simulink model "diff_drive_sim"  (Simulink 10.3)
settings: Solver=VariableStepAuto  StartTime=0.0  StopTime=30.1  RelTol=1e-3
values from neighbouring files (symbols this model uses):
  a = 4    [diff_drive.m]
  d = 0.1    [diff_drive.m]
  Kp = 1    [diff_drive.m]
  Kth = 2    [diff_drive.m]
  Kx = 15    [diff_drive.m]
  Ky = 15    [diff_drive.m]
  theta0 = pi/2    (= 1.57079632679)    [diff_drive.m]
  w = 0.1    [diff_drive.m]
  x0 = a    (= 4)    [diff_drive.m]
  y0 = 0    [diff_drive.m]
settings Model: Creator=olivier  LastModifiedBy=yukisaito  MultithreadedSim=on
settings SolverCC: ZeroCrossAlgorithm=Adaptive
settings DataIOCC: SaveFormat=Dataset  SignalLoggingSaveFormat=Dataset
settings OptimizationCC: ExpressionDepthLimit=128  LifeSpan=auto
settings DebuggingCC: UnderspecifiedInitializationDetection=Simplified  MergeDetectMultiDrivingBlocksExec=error  MaskedZcDiagnostic=none  IgnoredZcDiagnostic=none  FcnCallInpInsideContextMsg=error  StateNameClashWarn=none  SFUnexpectedBacktrackingDiag=error  SFNoUnconditionalDefaultTransitionDiag=error  SFExecutionAtInitializationDiag=warning
settings HardwareCC: ProdBitPerPointer=64  ProdBitPerSizeT=64  ProdBitPerPtrDiffT=64  ProdLargestAtomicFloat=Float  ProdIntDivRoundTo=Zero  ProdEndianess=LittleEndian  ProdWordSize=64  ProdHWDeviceType=Intel->x86-64 (Windows64)
settings ModelReferenceCC: PropagateSignalLabelsOutOfModel=on
settings SFSimCC: SimUseLocalCustomCode=on
settings RTWCC: RTWUseLocalCustomCode=on
settings CodeAppCC: StateflowObjectComments=off
settings GRTTargetCC: TargetLangStandard=C99 (ISO)  CombineOutputUpdateFcns=on  GRTInterface=off
settings ConfigComp: CovMetricSettings=dwe  CovSaveCumulativeToWorkspaceVar=off  CovSaveSingleToWorkspaceVar=off  CovExternalEMLEnable=on

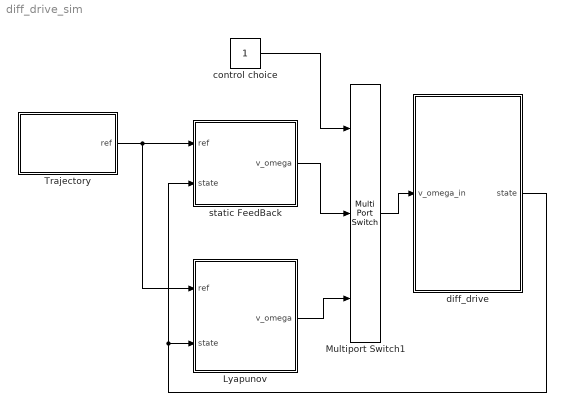
== system diff_drive_sim ==
  Lyapunov : Subsystem
  Multiport Switch1 : MultiPortSwitch  Inputs=2
  Trajectory : Subsystem  TreatAsAtomicUnit=on
  control choice : Constant
  diff_drive : Subsystem  mask{base=0.5, base_error=0, radius=0.2, radius_error=0, omega_max=80}
      mask prompts: base_error "Base error in percent"; radius_error "Radius error in percent"; omega_max "Wheel Max Velocity"
  static FeedBack : Subsystem
  wires:
  Trajectory/1(ref) -> Lyapunov/1(ref), static FeedBack/1(ref)
  Multiport Switch1/1 -> diff_drive/1(v_omega_in)
  control choice/1 -> Multiport Switch1/1
  diff_drive/1(state) -> static FeedBack/2(state), Lyapunov/2(state)
  static FeedBack/1(v_omega) -> Multiport Switch1/2
  Lyapunov/1(v_omega) -> Multiport Switch1/3

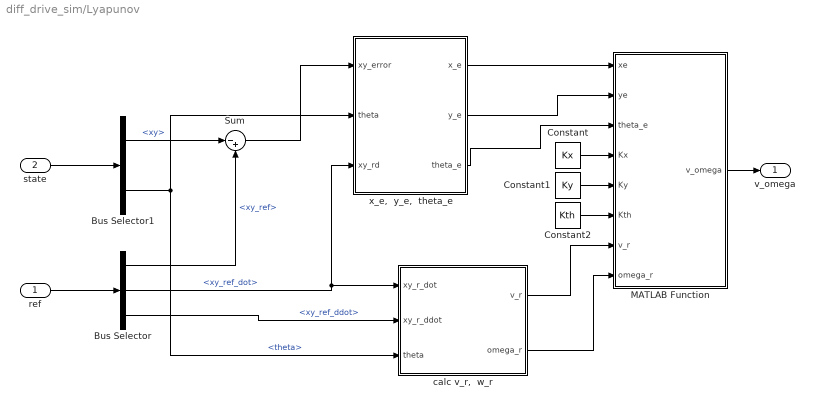
== system diff_drive_sim/Lyapunov ==
  ref : Inport
  state : Inport  Port=2
  Bus Selector : BusSelector  OutputSignals=xy_ref,xy_ref_dot,xy_ref_ddot
  Bus Selector1 : BusSelector  OutputSignals=xy,theta
  Constant : Constant  Value=Kx  VectorParams1D=off
  Constant1 : Constant  Value=Ky
  Constant2 : Constant  Value=Kth
  MATLAB Function : MATLAB Function  TreatAsAtomicUnit=on
  Sum : Sum  Inputs=|-+
  "calc v_r,  w_r" : MATLAB Function  TreatAsAtomicUnit=on
  "x_e,  y_e,  theta_e" : MATLAB Function  TreatAsAtomicUnit=on
  v_omega : Outport  VectorParamsAs1DForOutWhenUnconnected=off
  wires:
  ref/1 -> Bus Selector/1
  state/1 -> Bus Selector1/1
  Bus Selector/2 -> "x_e,  y_e,  theta_e"/3(xy_rd), "calc v_r,  w_r"/1(xy_r_dot)  "<xy_ref_dot>"
  Bus Selector/1 -> Sum/2  "<xy_ref>"
  Bus Selector/3 -> "calc v_r,  w_r"/2(xy_r_ddot)  "<xy_ref_ddot>"
  Bus Selector1/1 -> Sum/1  "<xy>"
  Bus Selector1/2 -> "x_e,  y_e,  theta_e"/2(theta), "calc v_r,  w_r"/3(theta)  "<theta>"
  Sum/1 -> "x_e,  y_e,  theta_e"/1(xy_error)
  MATLAB Function/1(v_omega) -> v_omega/1
  "x_e,  y_e,  theta_e"/1(x_e) -> MATLAB Function/1(xe)
  "x_e,  y_e,  theta_e"/2(y_e) -> MATLAB Function/2(ye)
  "x_e,  y_e,  theta_e"/3(theta_e) -> MATLAB Function/3(theta_e)
  "calc v_r,  w_r"/1(v_r) -> MATLAB Function/7(v_r)
  "calc v_r,  w_r"/2(omega_r) -> MATLAB Function/8(omega_r)
  Constant1/1 -> MATLAB Function/5(Ky)
  Constant/1 -> MATLAB Function/4(Kx)
  Constant2/1 -> MATLAB Function/6(Kth)

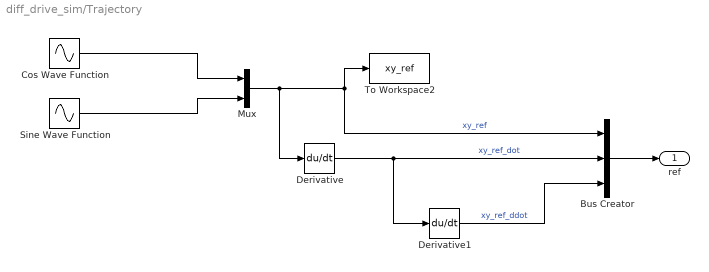
== system diff_drive_sim/Trajectory ==
  Bus Creator : BusCreator  Inputs=3
  Cos Wave Function : Sin  Amplitude=a  Frequency=w  Phase=pi/2  SampleTime=0
  Derivative : Derivative
  Derivative1 : Derivative
  Mux : Mux  Inputs=2
  Sine Wave Function : Sin  Amplitude=a  Frequency=w  SampleTime=0
  To Workspace2 : ToWorkspace  VariableName=xy_ref  SampleTime=-1
      settings: Save2DSignal=2-D array (concatenate along first dimension)
  ref : Outport  VectorParamsAs1DForOutWhenUnconnected=off
  wires:
  Bus Creator/1 -> ref/1
  Mux/1 -> Derivative/1, Bus Creator/1, To Workspace2/1  "xy_ref"
  Derivative/1 -> Bus Creator/2, Derivative1/1  "xy_ref_dot"
  Derivative1/1 -> Bus Creator/3  "xy_ref_ddot"
  Sine Wave Function/1 -> Mux/2
  Cos Wave Function/1 -> Mux/1

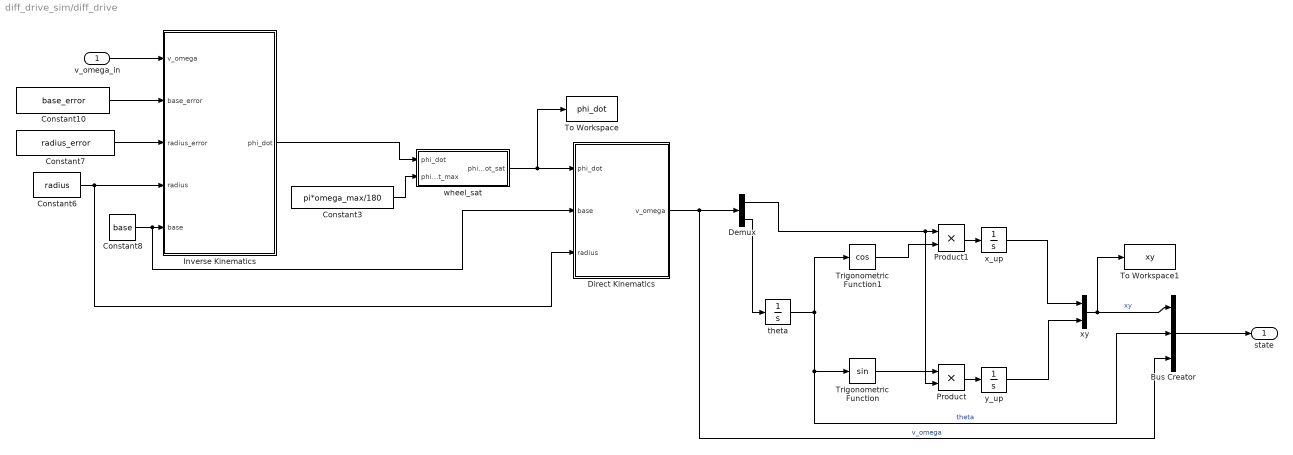
== system diff_drive_sim/diff_drive ==
  v_omega_in : Inport
  Bus Creator : BusCreator  Inputs=3
  Constant10 : Constant  Value=base_error
  Constant3 : Constant  Value=pi*omega_max/180
  Constant6 : Constant  Value=radius
  Constant7 : Constant  Value=radius_error
  Constant8 : Constant  Value=base
  Demux : Demux  Outputs=2
  Direct Kinematics : MATLAB Function  TreatAsAtomicUnit=on
  Inverse Kinematics : MATLAB Function  TreatAsAtomicUnit=on
  Product : Product
  Product1 : Product
  To Workspace : ToWorkspace  VariableName=phi_dot  SampleTime=-1
      settings: Save2DSignal=2-D array (concatenate along first dimension)
  To Workspace1 : ToWorkspace  VariableName=xy  SampleTime=-1
      settings: Save2DSignal=2-D array (concatenate along first dimension)
  Trigonometric Function : Trigonometry
  Trigonometric Function1 : Trigonometry  Operator=cos
  theta : Integrator  InitialCondition=theta0
  wheel_sat : Subsystem
  x_up : Integrator  InitialCondition=x0
  xy : Mux  Inputs=2
  y_up : Integrator  InitialCondition=y0
  state : Outport  VectorParamsAs1DForOutWhenUnconnected=off
  wires:
  theta/1 -> Trigonometric Function1/1, Trigonometric Function/1, Bus Creator/2  "theta"
  Trigonometric Function1/1 -> Product1/2
  Trigonometric Function/1 -> Product/1
  Product/1 -> y_up/1
  Product1/1 -> x_up/1
  x_up/1 -> xy/1
  Constant3/1 -> wheel_sat/2(phi_dot_max)
  Direct Kinematics/1(v_omega) -> Bus Creator/3, Demux/1  "v_omega"
  Demux/1 -> Product/2, Product1/1
  Demux/2 -> theta/1
  y_up/1 -> xy/2
  wheel_sat/1(phi_dot_sat) -> Direct Kinematics/1(phi_dot), To Workspace/1
  xy/1 -> Bus Creator/1, To Workspace1/1  "xy"
  Bus Creator/1 -> state/1
  Inverse Kinematics/1(phi_dot) -> wheel_sat/1(phi_dot)
  v_omega_in/1 -> Inverse Kinematics/1(v_omega)
  Constant10/1 -> Inverse Kinematics/2(base_error)
  Constant7/1 -> Inverse Kinematics/3(radius_error)
  Constant6/1 -> Inverse Kinematics/4(radius), Direct Kinematics/3(radius)
  Constant8/1 -> Direct Kinematics/2(base), Inverse Kinematics/5(base)

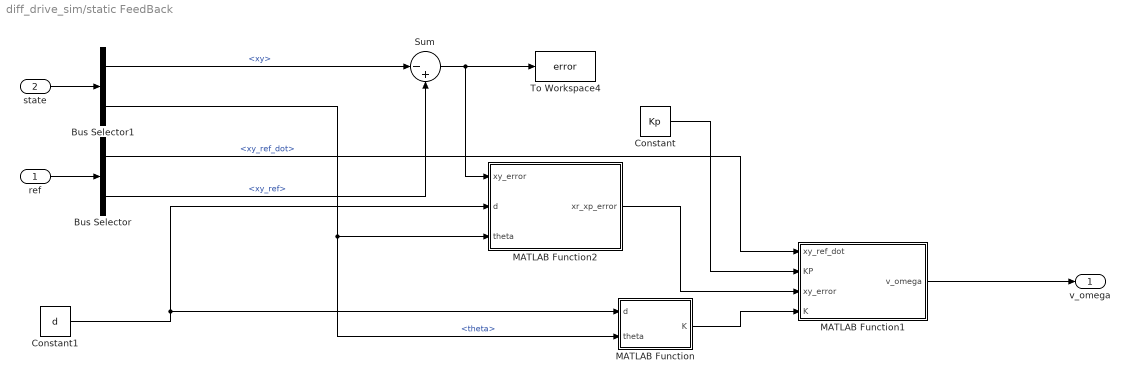
== system diff_drive_sim/static FeedBack ==
  ref : Inport
  state : Inport  Port=2
  Bus Selector : BusSelector  OutputSignals=xy_ref_dot,xy_ref
  Bus Selector1 : BusSelector  OutputSignals=xy,theta
  Constant : Constant  Value=Kp
  Constant1 : Constant  Value=d
  MATLAB Function : MATLAB Function  TreatAsAtomicUnit=on
  MATLAB Function1 : MATLAB Function  TreatAsAtomicUnit=on
  MATLAB Function2 : MATLAB Function  TreatAsAtomicUnit=on
  Sum : Sum  Inputs=|-+
  To Workspace4 : ToWorkspace  VariableName=error  SampleTime=-1
      settings: Save2DSignal=2-D array (concatenate along first dimension)
  v_omega : Outport  VectorParamsAs1DForOutWhenUnconnected=off
  wires:
  ref/1 -> Bus Selector/1
  state/1 -> Bus Selector1/1
  Bus Selector/2 -> Sum/2  "<xy_ref>"
  Bus Selector1/1 -> Sum/1  "<xy>"
  MATLAB Function1/1(v_omega) -> v_omega/1
  Bus Selector1/2 -> MATLAB Function/2(theta), MATLAB Function2/3(theta)  "<theta>"
  Bus Selector/1 -> MATLAB Function1/1(xy_ref_dot)  "<xy_ref_dot>"
  Constant1/1 -> MATLAB Function2/2(d), MATLAB Function/1(d)
  MATLAB Function/1(K) -> MATLAB Function1/4(K)
  Constant/1 -> MATLAB Function1/2(KP)
  MATLAB Function2/1(xr_xp_error) -> MATLAB Function1/3(xy_error)
  Sum/1 -> To Workspace4/1, MATLAB Function2/1(xy_error)

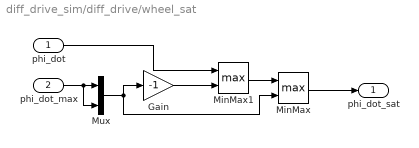
== system diff_drive_sim/diff_drive/wheel_sat ==
  phi_dot : Inport
  phi_dot_max : Inport  Port=2
  Gain : Gain  Gain=-1
  MinMax : MinMax  Function=max  Inputs=2
  MinMax1 : MinMax  Function=max  Inputs=2
  Mux : Mux  Inputs=2
  phi_dot_sat : Outport  VectorParamsAs1DForOutWhenUnconnected=off
  wires:
  Gain/1 -> MinMax1/2
  MinMax/1 -> phi_dot_sat/1
  phi_dot_max/1 -> Mux/2, Mux/1
  phi_dot/1 -> MinMax1/1
  MinMax1/1 -> MinMax/1
  Mux/1 -> MinMax/2, Gain/1

== matlab function diff_drive/Inverse Kinematics ==
  data: v_omega input double; base_error input double; radius_error input double; radius input double; phi_dot output double; base input double
function phi_dot = ik(v_omega, base_error, radius_error, radius, base)

base = base * (1+base_error*0.01);
radius = radius * (1+radius_error*0.01);

phi_dot = [(v_omega(1)+base*v_omega(2))/radius; (v_omega(1)-base*v_omega(2))/radius];

== matlab function static FeedBack/MATLAB Function ==
  data: d input double; K output double; theta input double
function K = fcn(d, theta)

K = [cos(theta) -d*sin(theta); sin(theta) d*cos(theta) ];

== matlab function static FeedBack/MATLAB Function1 ==
  data: xy_ref_dot input double; v_omega output double; KP input double; xy_error input double; K input double
function v_omega = fcn(xy_ref_dot, KP, xy_error, K)

Kp_error = KP*eye(2) * xy_error;
v_omega = inv(K)*(xy_ref_dot+Kp_error);

== matlab function diff_drive/Direct Kinematics ==
  data: phi_dot input double; v_omega output double; base input double; radius input double
function v_omega = dk(phi_dot, base, radius)

v_omega = [radius*(phi_dot(1)+phi_dot(2))/2; radius*(phi_dot(1)-phi_dot(2))/(2*base)];

== matlab function static FeedBack/MATLAB Function2 ==
  data: xy_error input double; xr_xp_error output double; d input double; theta input double
function xr_xp_error = fcn(xy_error, d, theta)

d_mat = [d*cos(theta); d*sin(theta)];

xr_xp_error = xy_error - d_mat;

== matlab function Lyapunov/calc v_r,  w_r ==
  data: xy_r_dot input double; v_r output double; xy_r_ddot input double; theta input double; omega_r output double
function [v_r, omega_r] = fcn(xy_r_dot, xy_r_ddot, theta)

v_r = xy_r_dot(1)*cos(theta)+xy_r_dot(2)*sin(theta);
if v_r == 0
    omega_r = 0;
else
    omega_r = (xy_r_dot(1)*xy_r_ddot(2) - xy_r_dot(2)*xy_r_ddot(1))/(v_r^2);
end

end

== matlab function Lyapunov/x_e,  y_e,  theta_e ==
  data: x_e output double; y_e output double; xy_error input double; theta input double; theta_e output double; xy_rd input double
function [x_e, y_e, theta_e]= fcn(xy_error, theta, xy_rd)
x_e = cos(theta)*xy_error(1)+sin(theta)*xy_error(2);
y_e = -sin(theta)*xy_error(1)+cos(theta)*xy_error(2);
theta_e = atan2(xy_rd(2), xy_rd(1)) - theta;
theta_e = theta_e - 2*pi * floor((theta_e+pi)/(2*pi));

== matlab function Lyapunov/MATLAB Function ==
  data: xe input double; v_omega output double; ye input double; theta_e input double; Kx input double; Ky input double; Kth input double; v_r input double; omega_r input double
function v_omega = fcn(xe, ye, theta_e, Kx, Ky, Kth, v_r, omega_r)
v = v_r*cos(theta_e)+Kx*xe;
omega = omega_r + (Ky*ye*v_r*sin(theta_e)/theta_e) + Kth*theta_e;
v_omega = [v; omega;];
%disp(size(v_omega));
